simulink model "SA_decouple_angles"  (R2016a)
settings: Solver=ode45  StartTime=0.0  StopTime=tfin  FixedStep=0.001  RelTol=1e-09
values from neighbouring files (symbols this model uses):
  den_av_SA91 = [1 -p_av_SA91]    [SA_9.m]    (also in SA_9cas1.m)
  den_AvPh_SA8 = [1 -p]    [SA_8.m]
  den_PI_SA8 = [1 -p]    [SA_8.m]
  den_re_SA91 = [1 -p_re_SA91]    [SA_9.m]    (also in SA_9cas1.m)
  Ka_av_SA91 = K_des/alf    [SA_9.m]    (also in SA_9cas1.m)
  Ka_SA8 = abs((polyval(den_phi,pdes)*polyval(den_AvPh_SA8,pdes)*polyval(den_PI_SA8,pdes))/(polyval(num_AvPh_SA8,pdes)*polyval(num_phi,pdes)*polyval(num_PI_SA8,pdes)))    [SA_8.m]
  Kp_XX = -z*Kv_XX    [SA_10.m]    (also in SA_10x.m; SA_10y.m)
  Kp_YY = -z*Kv_YY    [SA_10y.m]
  Kr_SA91 = K_des/beta    [SA_9.m]    (also in SA_9cas1.m)
  Kv_XX = 1/abs(polyval(conv(num_a_XX,num_Sx(1,:)),p_des)/polyval(conv(den_a_XX,den_Sx),p_des))    [SA_10.m]    (also in SA_10x.m; SA_10y.m)
  Kv_YY = 1/abs(polyval(conv(num_a_YY,num_Sy(1,:)),p_des)/polyval(conv(den_a_YY,den_Sy),p_des))    [SA_10y.m]
  num_av_SA91 = [1 -z_av_SA91]    [SA_9.m]    (also in SA_9cas1.m)
  num_AvPh_SA8 = [1 -z]    [SA_8.m]
  num_PI_SA8 = [1 -z]    [SA_8.m]
  num_re_SA91 = [1 -z_re_SA91]    [SA_9.m]    (also in SA_9cas1.m)
undefined symbols (not defined in the file or in its folder): A_phi, A_theta, A_z, ae0, ae1, ae2, ae3, as0, as1, as2, as3, AxS, AyS, B_phi, B_theta, B_z, be1, BxS, ByS, C3_3_iden, CxS, CyS, D_phi, D_theta, D_z, DxS, DyS, ia_e, ib_e, ic_e, phi_e, TABC_trans, TDEF_trans, theta_e, U, U_inv, va_e, vb_e, vc_e, vx_s_e, vy_s_e, vz_e, w_phi_e, w_theta_e, x_s_e, y_s_e, z_e
libraries: simulink_extras x3
settings Model: Creator=delafontaine  LastModifiedBy=genp2203
settings SolverCC: AlgebraicLoopSolver=LineSearch
settings DataIOCC: LimitDataPoints=on  SaveFormat=Array  SignalLoggingSaveFormat=ModelDataLogs
settings DebuggingCC: UnderspecifiedInitializationDetection=Classic  MergeDetectMultiDrivingBlocksExec=none  MultiTaskDSMMsg=warning  MultiTaskCondExecSysMsg=none
settings HardwareCC: ProdBitPerPointer=32  ProdLargestAtomicFloat=None  ProdIntDivRoundTo=Undefined  ProdEndianess=Unspecified  ProdWordSize=32  ProdHWDeviceType=32-bit Generic
settings ModelReferenceCC: PropagateSignalLabelsOutOfModel=off
settings ConfigComp: CovModelRefEnable=Off  CovSFcnEnable=off

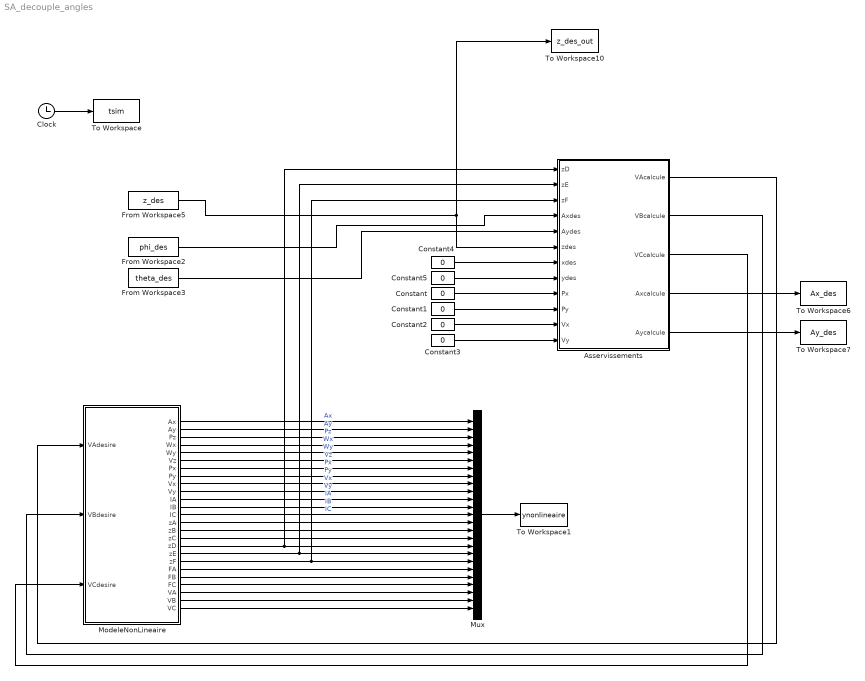
== system SA_decouple_angles ==
  Asservissements : Subsystem
      mask help: Simulink:masks:GenSFuncDesc_MD
      mask Help: eval('feval(''rtwprivate'',''rtwhelpview'',''rtw_sfcn_block'')');
  Clock : Clock
  Constant{,1..5} (6 alike) : Constant  Value=0
  From Workspace2 : FromWorkspace  VariableName=phi_des  SampleTime=0  Interpolate=off  OutputAfterFinalValue=Holding final value
  From Workspace3 : FromWorkspace  VariableName=theta_des  SampleTime=0  Interpolate=off  OutputAfterFinalValue=Holding final value
  From Workspace5 : FromWorkspace  VariableName=z_des  SampleTime=0  Interpolate=off  OutputAfterFinalValue=Holding final value
  ModeleNonLineaire : Subsystem
      mask help: Simulink:masks:GenSFuncDesc_MD
      mask Help: eval('feval(''rtwprivate'',''rtwhelpview'',''rtw_sfcn_block'')');
  Mux : Mux  Inputs=25
  To Workspace : ToWorkspace  VariableName=tsim  SampleTime=-1
  To Workspace1 : ToWorkspace  VariableName=ynonlineaire  SampleTime=-1
  To Workspace10 : ToWorkspace  VariableName=z_des_out  SampleTime=-1
  To Workspace6 : ToWorkspace  VariableName=Ax_des  SampleTime=-1
  To Workspace7 : ToWorkspace  VariableName=Ay_des  SampleTime=-1
  wires:
  Mux/1 -> To Workspace1/1
  Clock/1 -> To Workspace/1
  From Workspace5/1 -> Asservissements/6(zdes), To Workspace10/1
  ModeleNonLineaire/1(Ax) -> Mux/1  "Ax"
  ModeleNonLineaire/2(Ay) -> Mux/2  "Ay"
  ModeleNonLineaire/3(Pz) -> Mux/3  "Pz"
  ModeleNonLineaire/4(Wx) -> Mux/4  "Wx"
  ModeleNonLineaire/5(Wy) -> Mux/5  "Wy"
  ModeleNonLineaire/6(Vz) -> Mux/6  "Vz"
  ModeleNonLineaire/7(Px) -> Mux/7  "Px"
  ModeleNonLineaire/8(Py) -> Mux/8  "Py"
  ModeleNonLineaire/9(Vx) -> Mux/9  "Vx"
  ModeleNonLineaire/10(Vy) -> Mux/10  "Vy"
  ModeleNonLineaire/11(IA) -> Mux/11  "IA"
  ModeleNonLineaire/12(IB) -> Mux/12  "IB"
  ModeleNonLineaire/13(IC) -> Mux/13  "IC"
  ModeleNonLineaire/20(FA) -> Mux/20
  ModeleNonLineaire/21(FB) -> Mux/21
  ModeleNonLineaire/22(FC) -> Mux/22
  ModeleNonLineaire/23(VA) -> Mux/23
  ModeleNonLineaire/24(VB) -> Mux/24
  ModeleNonLineaire/25(VC) -> Mux/25
  ModeleNonLineaire/17(zD) -> Asservissements/1(zD), Mux/17
  ModeleNonLineaire/18(zE) -> Asservissements/2(zE), Mux/18
  ModeleNonLineaire/19(zF) -> Asservissements/3(zF), Mux/19
  ModeleNonLineaire/14(zA) -> Mux/14
  ModeleNonLineaire/15(zB) -> Mux/15
  ModeleNonLineaire/16(zC) -> Mux/16
  Asservissements/4(Axcalcule) -> To Workspace6/1
  Asservissements/5(Aycalcule) -> To Workspace7/1
  Asservissements/1(VAcalcule) -> ModeleNonLineaire/1(VAdesire)
  Asservissements/2(VBcalcule) -> ModeleNonLineaire/2(VBdesire)
  Asservissements/3(VCcalcule) -> ModeleNonLineaire/3(VCdesire)
  Constant/1 -> Asservissements/9(Px)
  Constant1/1 -> Asservissements/10(Py)
  Constant2/1 -> Asservissements/11(Vx)
  Constant3/1 -> Asservissements/12(Vy)
  From Workspace2/1 -> Asservissements/4(Axdes)
  From Workspace3/1 -> Asservissements/5(Aydes)
  Constant4/1 -> Asservissements/7(xdes)
  Constant5/1 -> Asservissements/8(ydes)

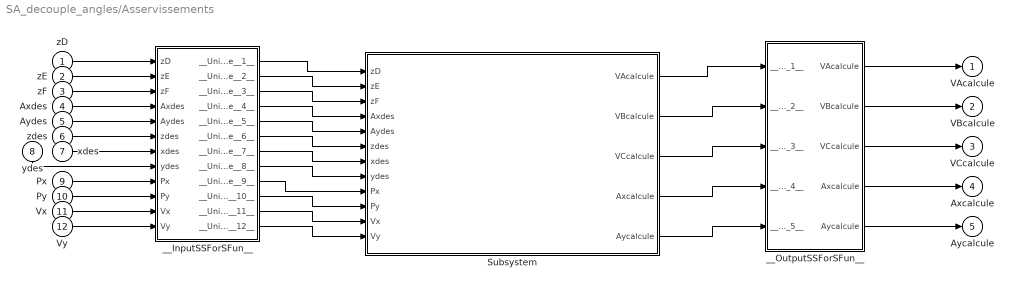
== system SA_decouple_angles/Asservissements ==
  zD : Inport
  zE : Inport  Port=2
  zF : Inport  Port=3
  Axdes : Inport  Port=4
  Aydes : Inport  Port=5
  zdes : Inport  Port=6
  xdes : Inport  Port=7
  ydes : Inport  Port=8
  Px : Inport  Port=9
  Py : Inport  Port=10
  Vx : Inport  Port=11
  Vy : Inport  Port=12
  Subsystem : Subsystem
  __InputSSForSFun__ : Subsystem
  __OutputSSForSFun__ : Subsystem
  VAcalcule : Outport
  VBcalcule : Outport  Port=2
  VCcalcule : Outport  Port=3
  Axcalcule : Outport  Port=4
  Aycalcule : Outport  Port=5
  wires:
  zD/1 -> __InputSSForSFun__/1(zD)
  zE/1 -> __InputSSForSFun__/2(zE)
  zF/1 -> __InputSSForSFun__/3(zF)
  Axdes/1 -> __InputSSForSFun__/4(Axdes)
  Aydes/1 -> __InputSSForSFun__/5(Aydes)
  zdes/1 -> __InputSSForSFun__/6(zdes)
  xdes/1 -> __InputSSForSFun__/7(xdes)
  ydes/1 -> __InputSSForSFun__/8(ydes)
  Px/1 -> __InputSSForSFun__/9(Px)
  Py/1 -> __InputSSForSFun__/10(Py)
  Vx/1 -> __InputSSForSFun__/11(Vx)
  Vy/1 -> __InputSSForSFun__/12(Vy)
  __InputSSForSFun__/1(__UniqueOutportName__1__) -> Subsystem/1(zD)
  __InputSSForSFun__/2(__UniqueOutportName__2__) -> Subsystem/2(zE)
  __InputSSForSFun__/3(__UniqueOutportName__3__) -> Subsystem/3(zF)
  __InputSSForSFun__/4(__UniqueOutportName__4__) -> Subsystem/4(Axdes)
  __InputSSForSFun__/5(__UniqueOutportName__5__) -> Subsystem/5(Aydes)
  __InputSSForSFun__/6(__UniqueOutportName__6__) -> Subsystem/6(zdes)
  __InputSSForSFun__/7(__UniqueOutportName__7__) -> Subsystem/7(xdes)
  __InputSSForSFun__/8(__UniqueOutportName__8__) -> Subsystem/8(ydes)
  __InputSSForSFun__/9(__UniqueOutportName__9__) -> Subsystem/9(Px)
  __InputSSForSFun__/10(__UniqueOutportName__10__) -> Subsystem/10(Py)
  __InputSSForSFun__/11(__UniqueOutportName__11__) -> Subsystem/11(Vx)
  __InputSSForSFun__/12(__UniqueOutportName__12__) -> Subsystem/12(Vy)
  Subsystem/1(VAcalcule) -> __OutputSSForSFun__/1(__UniqueInportName__1__)
  Subsystem/2(VBcalcule) -> __OutputSSForSFun__/2(__UniqueInportName__2__)
  Subsystem/3(VCcalcule) -> __OutputSSForSFun__/3(__UniqueInportName__3__)
  Subsystem/4(Axcalcule) -> __OutputSSForSFun__/4(__UniqueInportName__4__)
  Subsystem/5(Aycalcule) -> __OutputSSForSFun__/5(__UniqueInportName__5__)
  __OutputSSForSFun__/1(VAcalcule) -> VAcalcule/1
  __OutputSSForSFun__/2(VBcalcule) -> VBcalcule/1
  __OutputSSForSFun__/3(VCcalcule) -> VCcalcule/1
  __OutputSSForSFun__/4(Axcalcule) -> Axcalcule/1
  __OutputSSForSFun__/5(Aycalcule) -> Aycalcule/1

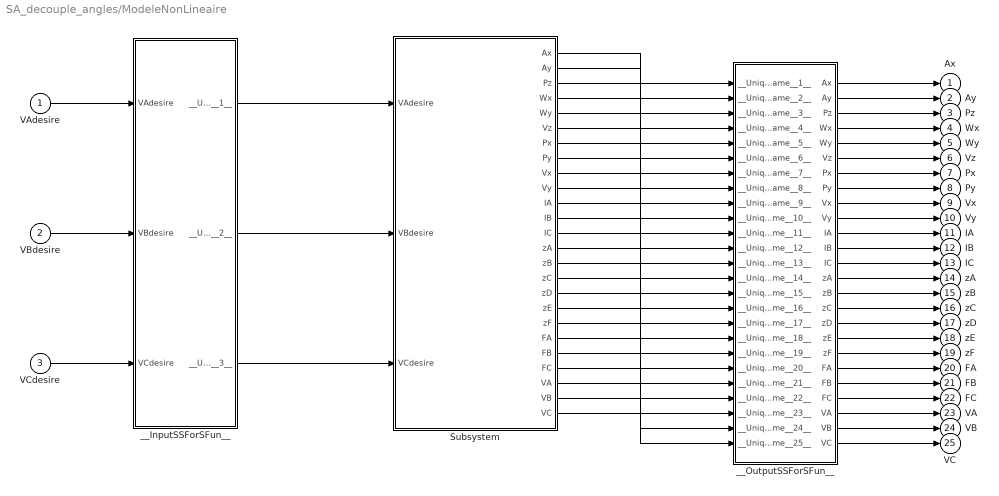
== system SA_decouple_angles/ModeleNonLineaire ==
  VAdesire : Inport
  VBdesire : Inport  Port=2
  VCdesire : Inport  Port=3
  Subsystem : Subsystem
  __InputSSForSFun__ : Subsystem
  __OutputSSForSFun__ : Subsystem
  Ax : Outport
  Ay : Outport  Port=2
  Pz : Outport  Port=3
  Wx : Outport  Port=4
  Wy : Outport  Port=5
  Vz : Outport  Port=6
  Px : Outport  Port=7
  Py : Outport  Port=8
  Vx : Outport  Port=9
  Vy : Outport  Port=10
  IA : Outport  Port=11
  IB : Outport  Port=12
  IC : Outport  Port=13
  zA : Outport  Port=14
  zB : Outport  Port=15
  zC : Outport  Port=16
  zD : Outport  Port=17
  zE : Outport  Port=18
  zF : Outport  Port=19
  FA : Outport  Port=20
  FB : Outport  Port=21
  FC : Outport  Port=22
  VA : Outport  Port=23
  VB : Outport  Port=24
  VC : Outport  Port=25
  wires:
  VAdesire/1 -> __InputSSForSFun__/1(VAdesire)
  VBdesire/1 -> __InputSSForSFun__/2(VBdesire)
  VCdesire/1 -> __InputSSForSFun__/3(VCdesire)
  __InputSSForSFun__/1(__UniqueOutportName__1__) -> Subsystem/1(VAdesire)
  __InputSSForSFun__/2(__UniqueOutportName__2__) -> Subsystem/2(VBdesire)
  __InputSSForSFun__/3(__UniqueOutportName__3__) -> Subsystem/3(VCdesire)
  Subsystem/1(Ax) -> __OutputSSForSFun__/1(__UniqueInportName__1__)
  Subsystem/2(Ay) -> __OutputSSForSFun__/2(__UniqueInportName__2__)
  Subsystem/3(Pz) -> __OutputSSForSFun__/3(__UniqueInportName__3__)
  Subsystem/4(Wx) -> __OutputSSForSFun__/4(__UniqueInportName__4__)
  Subsystem/5(Wy) -> __OutputSSForSFun__/5(__UniqueInportName__5__)
  Subsystem/6(Vz) -> __OutputSSForSFun__/6(__UniqueInportName__6__)
  Subsystem/7(Px) -> __OutputSSForSFun__/7(__UniqueInportName__7__)
  Subsystem/8(Py) -> __OutputSSForSFun__/8(__UniqueInportName__8__)
  Subsystem/9(Vx) -> __OutputSSForSFun__/9(__UniqueInportName__9__)
  Subsystem/10(Vy) -> __OutputSSForSFun__/10(__UniqueInportName__10__)
  Subsystem/11(IA) -> __OutputSSForSFun__/11(__UniqueInportName__11__)
  Subsystem/12(IB) -> __OutputSSForSFun__/12(__UniqueInportName__12__)
  Subsystem/13(IC) -> __OutputSSForSFun__/13(__UniqueInportName__13__)
  Subsystem/14(zA) -> __OutputSSForSFun__/14(__UniqueInportName__14__)
  Subsystem/15(zB) -> __OutputSSForSFun__/15(__UniqueInportName__15__)
  Subsystem/16(zC) -> __OutputSSForSFun__/16(__UniqueInportName__16__)
  Subsystem/17(zD) -> __OutputSSForSFun__/17(__UniqueInportName__17__)
  Subsystem/18(zE) -> __OutputSSForSFun__/18(__UniqueInportName__18__)
  Subsystem/19(zF) -> __OutputSSForSFun__/19(__UniqueInportName__19__)
  Subsystem/20(FA) -> __OutputSSForSFun__/20(__UniqueInportName__20__)
  Subsystem/21(FB) -> __OutputSSForSFun__/21(__UniqueInportName__21__)
  Subsystem/22(FC) -> __OutputSSForSFun__/22(__UniqueInportName__22__)
  Subsystem/23(VA) -> __OutputSSForSFun__/23(__UniqueInportName__23__)
  Subsystem/24(VB) -> __OutputSSForSFun__/24(__UniqueInportName__24__)
  Subsystem/25(VC) -> __OutputSSForSFun__/25(__UniqueInportName__25__)
  __OutputSSForSFun__/1(Ax) -> Ax/1
  __OutputSSForSFun__/2(Ay) -> Ay/1
  __OutputSSForSFun__/3(Pz) -> Pz/1
  __OutputSSForSFun__/4(Wx) -> Wx/1
  __OutputSSForSFun__/5(Wy) -> Wy/1
  __OutputSSForSFun__/6(Vz) -> Vz/1
  __OutputSSForSFun__/7(Px) -> Px/1
  __OutputSSForSFun__/8(Py) -> Py/1
  __OutputSSForSFun__/9(Vx) -> Vx/1
  __OutputSSForSFun__/10(Vy) -> Vy/1
  __OutputSSForSFun__/11(IA) -> IA/1
  __OutputSSForSFun__/12(IB) -> IB/1
  __OutputSSForSFun__/13(IC) -> IC/1
  __OutputSSForSFun__/14(zA) -> zA/1
  __OutputSSForSFun__/15(zB) -> zB/1
  __OutputSSForSFun__/16(zC) -> zC/1
  __OutputSSForSFun__/17(zD) -> zD/1
  __OutputSSForSFun__/18(zE) -> zE/1
  __OutputSSForSFun__/19(zF) -> zF/1
  __OutputSSForSFun__/20(FA) -> FA/1
  __OutputSSForSFun__/21(FB) -> FB/1
  __OutputSSForSFun__/22(FC) -> FC/1
  __OutputSSForSFun__/23(VA) -> VA/1
  __OutputSSForSFun__/24(VB) -> VB/1
  __OutputSSForSFun__/25(VC) -> VC/1

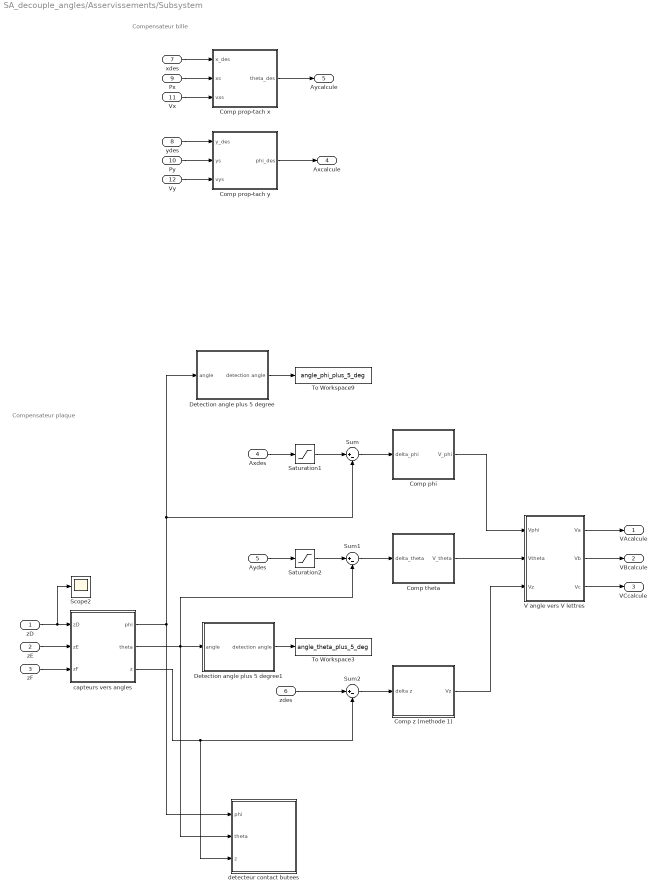
== system SA_decouple_angles/Asservissements/Subsystem ==
  note: Compensateur plaque
  note: Compensateur bille
  zD : Inport
  zE : Inport  Port=2
  zF : Inport  Port=3
  Axdes : Inport  Port=4
  Aydes : Inport  Port=5
  zdes : Inport  Port=6
  xdes : Inport  Port=7
  ydes : Inport  Port=8
  Px : Inport  Port=9
  Py : Inport  Port=10
  Vx : Inport  Port=11
  Vy : Inport  Port=12
  Comp phi : Subsystem
  Comp prop-tach x : Subsystem
  Comp prop-tach y : Subsystem
  Comp theta : Subsystem
  Comp z (methode 1) : Subsystem
  Detection angle plus 5 degree : Subsystem
  Detection angle plus 5 degree1 : Subsystem
  Saturation1 : Saturate  UpperLimit=deg2rad(5)  LowerLimit=deg2rad(-5)
  Saturation2 : Saturate  UpperLimit=deg2rad(5)  LowerLimit=deg2rad(-5)
  Scope2 : Scope
  Sum : Sum  Inputs=|+-
  Sum1 : Sum  Inputs=|+-
  Sum2 : Sum  Inputs=|+-
  To Workspace3 : ToWorkspace  VariableName=angle_theta_plus_5_deg  SampleTime=-1
      settings: MaxDataPoints=1
  To Workspace9 : ToWorkspace  VariableName=angle_phi_plus_5_deg  SampleTime=-1
      settings: MaxDataPoints=1
  V angle vers V lettres : Subsystem
  capteurs vers angles : Subsystem
  detecteur contact butees : Subsystem
  VAcalcule : Outport
  VBcalcule : Outport  Port=2
  VCcalcule : Outport  Port=3
  Axcalcule : Outport  Port=4
  Aycalcule : Outport  Port=5
  wires:
  Sum/1 -> Comp phi/1(delta_phi)
  ydes/1 -> Comp prop-tach y/1(y_des)
  xdes/1 -> Comp prop-tach x/1(x_des)
  Vx/1 -> Comp prop-tach x/3(vxs)
  Px/1 -> Comp prop-tach x/2(xs)
  Py/1 -> Comp prop-tach y/2(ys)
  Vy/1 -> Comp prop-tach y/3(vys)
  zD/1 -> Scope2/1, capteurs vers angles/1(zD)
  zE/1 -> capteurs vers angles/2(zE)
  zF/1 -> capteurs vers angles/3(zF)
  capteurs vers angles/1(phi) -> Sum/2, Detection angle plus 5 degree/1(angle), detecteur contact butees/1(phi)
  V angle vers V lettres/3(Vc) -> VCcalcule/1
  V angle vers V lettres/2(Vb) -> VBcalcule/1
  V angle vers V lettres/1(Va) -> VAcalcule/1
  Comp phi/1(V_phi) -> V angle vers V lettres/1(Vphi)
  Comp theta/1(V_theta) -> V angle vers V lettres/2(Vtheta)
  Sum1/1 -> Comp theta/1(delta_theta)
  capteurs vers angles/3(z) -> detecteur contact butees/3(z), Sum2/2
  zdes/1 -> Sum2/1
  Sum2/1 -> Comp z (methode 1)/1(delta z)
  Comp prop-tach y/1(phi_des) -> Axcalcule/1
  Comp prop-tach x/1(theta_des) -> Aycalcule/1
  Comp z (methode 1)/1(Vz) -> V angle vers V lettres/3(Vz)
  Detection angle plus 5 degree/1(detection angle) -> To Workspace9/1
  Detection angle plus 5 degree1/1(detection angle) -> To Workspace3/1
  capteurs vers angles/2(theta) -> Detection angle plus 5 degree1/1(angle), Sum1/2, detecteur contact butees/2(theta)
  Axdes/1 -> Saturation1/1
  Saturation1/1 -> Sum/1
  Saturation2/1 -> Sum1/1
  Aydes/1 -> Saturation2/1

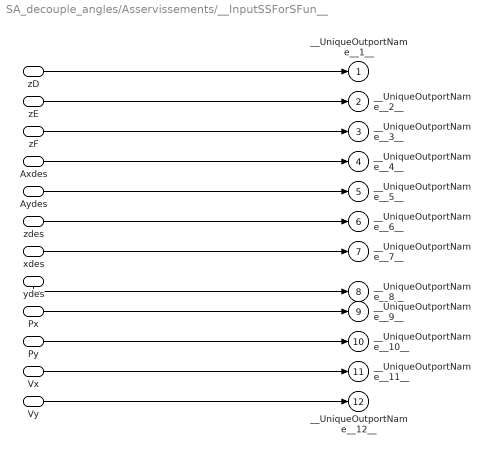
== system SA_decouple_angles/Asservissements/__InputSSForSFun__ ==
  zD : Inport
  zE : Inport  Port=2
  zF : Inport  Port=3
  Axdes : Inport  Port=4
  Aydes : Inport  Port=5
  zdes : Inport  Port=6
  xdes : Inport  Port=7
  ydes : Inport  Port=8
  Px : Inport  Port=9
  Py : Inport  Port=10
  Vx : Inport  Port=11
  Vy : Inport  Port=12
  __UniqueOutportName__1__ : Outport
  __UniqueOutportName__2__ : Outport  Port=2
  __UniqueOutportName__3__ : Outport  Port=3
  __UniqueOutportName__4__ : Outport  Port=4
  __UniqueOutportName__5__ : Outport  Port=5
  __UniqueOutportName__6__ : Outport  Port=6
  __UniqueOutportName__7__ : Outport  Port=7
  __UniqueOutportName__8__ : Outport  Port=8
  __UniqueOutportName__9__ : Outport  Port=9
  __UniqueOutportName__10__ : Outport  Port=10
  __UniqueOutportName__11__ : Outport  Port=11
  __UniqueOutportName__12__ : Outport  Port=12
  wires:
  zD/1 -> __UniqueOutportName__1__/1
  zE/1 -> __UniqueOutportName__2__/1
  zF/1 -> __UniqueOutportName__3__/1
  Axdes/1 -> __UniqueOutportName__4__/1
  Aydes/1 -> __UniqueOutportName__5__/1
  zdes/1 -> __UniqueOutportName__6__/1
  xdes/1 -> __UniqueOutportName__7__/1
  ydes/1 -> __UniqueOutportName__8__/1
  Px/1 -> __UniqueOutportName__9__/1
  Py/1 -> __UniqueOutportName__10__/1
  Vx/1 -> __UniqueOutportName__11__/1
  Vy/1 -> __UniqueOutportName__12__/1

== system SA_decouple_angles/Asservissements/__OutputSSForSFun__ ==
  __UniqueInportName__1__ : Inport
  __UniqueInportName__2__ : Inport  Port=2
  __UniqueInportName__3__ : Inport  Port=3
  __UniqueInportName__4__ : Inport  Port=4
  __UniqueInportName__5__ : Inport  Port=5
  VAcalcule : Outport
  VBcalcule : Outport  Port=2
  VCcalcule : Outport  Port=3
  Axcalcule : Outport  Port=4
  Aycalcule : Outport  Port=5
  wires:
  __UniqueInportName__1__/1 -> VAcalcule/1
  __UniqueInportName__2__/1 -> VBcalcule/1
  __UniqueInportName__3__/1 -> VCcalcule/1
  __UniqueInportName__4__/1 -> Axcalcule/1  "Ax_des"
  __UniqueInportName__5__/1 -> Aycalcule/1  "Ay_des"

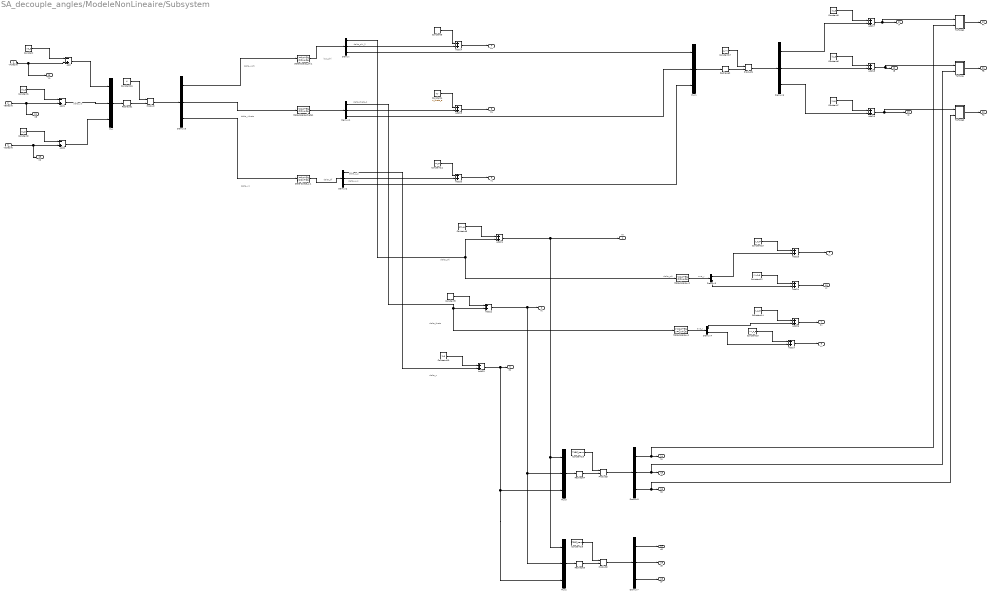
== system SA_decouple_angles/ModeleNonLineaire/Subsystem ==
  note: axe_x
  note: axe_y
  note: delta_phi
  note: delta_w_z
  note: delta_z_2
  note: delta_theta_2
  note: delta_phi_2
  note: delta_phi
  note: delta_vb
  note: delta_z
  note: delta_theta
  note: bus_phi
  note: delat_df
  note: delta_vphi
  note: delta_vtheta
  note: delta_vz
  VAdesire : Inport
  VBdesire : Inport  Port=2
  VCdesire : Inport  Port=3
  Add : Sum  Inputs=-+
  Add1 : Sum  Inputs=-+
  Add{13..14,17..27} (13 alike) : Sum
  Add2 : Sum  Inputs=-+
  Constant : Constant  Value=va_e
  Constant1 : Constant  Value=vb_e
  Constant10 : Constant  Value=z_e
  Constant11 : Constant  Value=vz_e
  Constant12 : Constant  Value=vy_s_e
  Constant13 : Constant  Value=y_s_e
  Constant14 : Constant  Value=x_s_e
  Constant15 : Constant  Value=vx_s_e
  Constant16 : Constant  Value=U  VectorParams1D=off
  Constant17 : Constant  Value=U_inv  VectorParams1D=off
  Constant18 : Constant  Value=TDEF_trans  VectorParams1D=off
  Constant19 : Constant  Value=TABC_trans  VectorParams1D=off
  Constant2 : Constant  Value=vc_e
  Constant3 : Constant  Value=ia_e
  Constant4 : Constant  Value=w_theta_e
  Constant5 : Constant  Value=w_phi_e
  Constant6 : Constant  Value=ib_e
  Constant7 : Constant  Value=ic_e
  Constant8 : Constant  Value=phi_e
  Constant9 : Constant  Value=theta_e
  Demux{,1..2,5..8} (7 alike) : Demux  Outputs=3
  Demux3 : Demux  Outputs=2
  Demux4 : Demux  Outputs=2
  Mux{,1..3} (4 alike) : Mux  Inputs=3
  Product{,1..3} (4 alike) : Product  Multiplication=Matrix(*)
  Reshape{1..4} (4 alike) : Reshape  OutputDimensionality=Column vector (2-D)  OutputDimensions=[3:1]
  State-Space_phi1 : StateSpace  A=A_phi  B=B_phi  C=C3_3_iden  D=D_phi  X0=0
  State-Space_theta1 : StateSpace  A=A_theta  B=B_theta  C=C3_3_iden  D=D_theta  X0=0
  State-Space_xs : StateSpace  A=AyS  B=ByS  C=CyS  D=DyS  X0=0
  State-Space_ys : StateSpace  A=AxS  B=BxS  C=CxS  D=DxS  X0=0
  State-Space_z 1 : StateSpace  A=A_z  B=B_z  C=C3_3_iden  D=D_z  X0=0
  ToForce : Subsystem
  ToForce1 : Subsystem
  ToForce2 : Subsystem
  Ax : Outport
  Ay : Outport  Port=2
  Pz : Outport  Port=3
  Wx : Outport  Port=4
  Wy : Outport  Port=5
  Vz : Outport  Port=6
  Px : Outport  Port=7
  Py : Outport  Port=8
  Vx : Outport  Port=9
  Vy : Outport  Port=10
  IA : Outport  Port=11
  IB : Outport  Port=12
  IC : Outport  Port=13
  zA : Outport  Port=14
  zB : Outport  Port=15
  zC : Outport  Port=16
  zD : Outport  Port=17
  zE : Outport  Port=18
  zF : Outport  Port=19
  FA : Outport  Port=20
  FB : Outport  Port=21
  FC : Outport  Port=22
  VA : Outport  Port=23
  VB : Outport  Port=24
  VC : Outport  Port=25
  wires:
  Constant/1 -> Add/1
  VAdesire/1 -> VA/1, Add/2
  Constant2/1 -> Add2/1
  VCdesire/1 -> VC/1, Add2/2
  Constant1/1 -> Add1/1
  VBdesire/1 -> VB/1, Add1/2
  Demux2/1 -> Add23/2
  Demux5/1 -> State-Space_phi1/1
  Demux5/2 -> State-Space_theta1/1
  Demux5/3 -> State-Space_z 1/1
  State-Space_phi1/1 -> Demux/1
  State-Space_theta1/1 -> Demux1/1  "delta_de"
  State-Space_z 1/1 -> Demux2/1
  Demux1/2 -> Add13/2  "delta_w_theta"
  Demux2/2 -> Add20/2
  Constant4/1 -> Add13/1
  Constant5/1 -> Add14/1
  Constant11/1 -> Add20/1
  Add14/1 -> Wx/1
  Add13/1 -> Wy/1
  Add20/1 -> Vz/1
  Demux/3 -> Mux1/1  "delta_i_phi"
  Demux1/3 -> Mux1/2  "delta_i_theta"
  Demux2/3 -> Mux1/3  "delta_i_z"
  Constant3/1 -> Add17/1
  Constant6/1 -> Add18/1
  Constant7/1 -> Add19/1
  Constant8/1 -> Add21/1
  Constant9/1 -> Add22/1
  Constant10/1 -> Add23/1
  Demux/1 -> Add21/2, State-Space_xs/1
  State-Space_xs/1 -> Demux3/1
  Demux1/1 -> State-Space_ys/1, Add22/2  "delta_theta"
  State-Space_ys/1 -> Demux4/1
  Demux3/1 -> Add25/2  "delta_ys"
  Demux3/2 -> Add24/2  "dela_vys"
  Demux4/1 -> Add26/2  "delta_xs"
  Demux4/2 -> Add27/2  "delta_vxs"
  Constant12/1 -> Add24/1
  Constant13/1 -> Add25/1
  Constant14/1 -> Add26/1
  Constant15/1 -> Add27/1
  Add25/1 -> Py/1
  Add24/1 -> Vy/1
  Add26/1 -> Px/1
  Add27/1 -> Vx/1
  Demux7/1 -> zD/1
  Add21/1 -> Mux3/1, Mux2/1, Ax/1  "phi"
  Demux7/2 -> zE/1
  Add22/1 -> Mux3/2, Mux2/2, Ay/1  "theta"
  Add23/1 -> Mux3/3, Mux2/3, Pz/1  "z"
  Demux7/3 -> zF/1
  Add17/1 -> ToForce1/1(I), IA/1
  Add18/1 -> IB/1, ToForce/1(I)
  Add19/1 -> ToForce2/1(I), IC/1
  ToForce/1(Force) -> FB/1
  ToForce1/1(Force) -> FA/1
  ToForce2/1(Force) -> FC/1
  Add/1 -> Mux/1  "delta_va"
  Add1/1 -> Mux/2  "delta_vb"
  Add2/1 -> Mux/3  "delta_vc"
  Constant16/1 -> Product/1
  Product/1 -> Demux5/1
  Mux/1 -> Reshape1/1
  Reshape1/1 -> Product/2
  Constant17/1 -> Product1/1
  Product1/1 -> Demux6/1
  Mux1/1 -> Reshape2/1
  Reshape2/1 -> Product1/2
  Demux6/1 -> Add17/2
  Demux6/2 -> Add18/2
  Demux6/3 -> Add19/2
  Demux/2 -> Add14/2  "delta_w_phi"
  Constant18/1 -> Product2/1
  Product2/1 -> Demux7/1
  Mux2/1 -> Reshape3/1
  Reshape3/1 -> Product2/2
  Constant19/1 -> Product3/1
  Product3/1 -> Demux8/1
  Mux3/1 -> Reshape4/1
  Reshape4/1 -> Product3/2
  Demux8/3 -> ToForce2/2(Z), zC/1
  Demux8/2 -> zB/1, ToForce/2(Z)
  Demux8/1 -> ToForce1/2(Z), zA/1

== system SA_decouple_angles/ModeleNonLineaire/__InputSSForSFun__ ==
  VAdesire : Inport
  VBdesire : Inport  Port=2
  VCdesire : Inport  Port=3
  __UniqueOutportName__1__ : Outport
  __UniqueOutportName__2__ : Outport  Port=2
  __UniqueOutportName__3__ : Outport  Port=3
  wires:
  VAdesire/1 -> __UniqueOutportName__1__/1
  VBdesire/1 -> __UniqueOutportName__2__/1
  VCdesire/1 -> __UniqueOutportName__3__/1

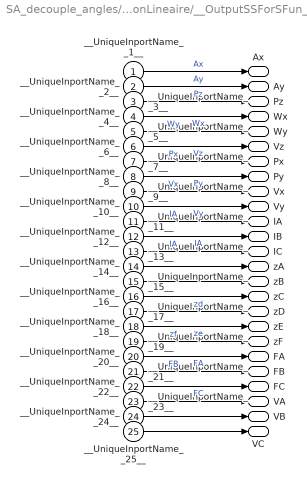
== system SA_decouple_angles/ModeleNonLineaire/__OutputSSForSFun__ ==
  __UniqueInportName__1__ : Inport
  __UniqueInportName__2__ : Inport  Port=2
  __UniqueInportName__3__ : Inport  Port=3
  __UniqueInportName__4__ : Inport  Port=4
  __UniqueInportName__5__ : Inport  Port=5
  __UniqueInportName__6__ : Inport  Port=6
  __UniqueInportName__7__ : Inport  Port=7
  __UniqueInportName__8__ : Inport  Port=8
  __UniqueInportName__9__ : Inport  Port=9
  __UniqueInportName__10__ : Inport  Port=10
  __UniqueInportName__11__ : Inport  Port=11
  __UniqueInportName__12__ : Inport  Port=12
  __UniqueInportName__13__ : Inport  Port=13
  __UniqueInportName__14__ : Inport  Port=14
  __UniqueInportName__15__ : Inport  Port=15
  __UniqueInportName__16__ : Inport  Port=16
  __UniqueInportName__17__ : Inport  Port=17
  __UniqueInportName__18__ : Inport  Port=18
  __UniqueInportName__19__ : Inport  Port=19
  __UniqueInportName__20__ : Inport  Port=20
  __UniqueInportName__21__ : Inport  Port=21
  __UniqueInportName__22__ : Inport  Port=22
  __UniqueInportName__23__ : Inport  Port=23
  __UniqueInportName__24__ : Inport  Port=24
  __UniqueInportName__25__ : Inport  Port=25
  Ax : Outport
  Ay : Outport  Port=2
  Pz : Outport  Port=3
  Wx : Outport  Port=4
  Wy : Outport  Port=5
  Vz : Outport  Port=6
  Px : Outport  Port=7
  Py : Outport  Port=8
  Vx : Outport  Port=9
  Vy : Outport  Port=10
  IA : Outport  Port=11
  IB : Outport  Port=12
  IC : Outport  Port=13
  zA : Outport  Port=14
  zB : Outport  Port=15
  zC : Outport  Port=16
  zD : Outport  Port=17
  zE : Outport  Port=18
  zF : Outport  Port=19
  FA : Outport  Port=20
  FB : Outport  Port=21
  FC : Outport  Port=22
  VA : Outport  Port=23
  VB : Outport  Port=24
  VC : Outport  Port=25
  wires:
  __UniqueInportName__1__/1 -> Ax/1  "Ax"
  __UniqueInportName__2__/1 -> Ay/1  "Ay"
  __UniqueInportName__3__/1 -> Pz/1  "Pz"
  __UniqueInportName__4__/1 -> Wx/1  "Wx"
  __UniqueInportName__5__/1 -> Wy/1  "Wy"
  __UniqueInportName__6__/1 -> Vz/1  "Vz"
  __UniqueInportName__7__/1 -> Px/1  "Px"
  __UniqueInportName__8__/1 -> Py/1  "Py"
  __UniqueInportName__9__/1 -> Vx/1  "Vx"
  __UniqueInportName__10__/1 -> Vy/1  "Vy"
  __UniqueInportName__11__/1 -> IA/1  "IA"
  __UniqueInportName__12__/1 -> IB/1  "IA"
  __UniqueInportName__13__/1 -> IC/1  "IA"
  __UniqueInportName__14__/1 -> zA/1
  __UniqueInportName__15__/1 -> zB/1
  __UniqueInportName__16__/1 -> zC/1
  __UniqueInportName__17__/1 -> zD/1  "zd"
  __UniqueInportName__18__/1 -> zE/1  "ze"
  __UniqueInportName__19__/1 -> zF/1  "zf"
  __UniqueInportName__20__/1 -> FA/1  "FA"
  __UniqueInportName__21__/1 -> FB/1  "FB"
  __UniqueInportName__22__/1 -> FC/1  "FC"
  __UniqueInportName__23__/1 -> VA/1
  __UniqueInportName__24__/1 -> VB/1
  __UniqueInportName__25__/1 -> VC/1

== system SA_decouple_angles/Asservissements/Subsystem/Comp phi ==
  delta_phi : Inport
  Double_AvPh : Subsystem
  PI : TransferFcn  Numerator=num_PI_SA8  Denominator=den_PI_SA8
  V_phi : Outport
  wires:
  PI/1 -> Double_AvPh/1(signal_in)
  delta_phi/1 -> PI/1
  Double_AvPh/1(signal_out) -> V_phi/1

== system SA_decouple_angles/Asservissements/Subsystem/Comp prop-tach x ==
  x_des : Inport
  xs : Inport  Port=2
  vxs : Inport  Port=3
  Gain : Gain  Gain=Kv_XX
  Gain1 : Gain  Gain=Kp_XX
  Sum : Sum  Inputs=|-+
  Sum1 : Sum  Inputs=|++
  theta_des : Outport
  wires:
  Sum/1 -> Gain1/1
  Gain1/1 -> Sum1/1
  Gain/1 -> Sum1/2
  xs/1 -> Sum/2
  vxs/1 -> Gain/1
  Sum1/1 -> theta_des/1
  x_des/1 -> Sum/1

== system SA_decouple_angles/Asservissements/Subsystem/Comp prop-tach y ==
  y_des : Inport
  ys : Inport  Port=2
  vys : Inport  Port=3
  Gain : Gain  Gain=Kv_YY
  Gain1 : Gain  Gain=Kp_YY
  Sum : Sum  Inputs=|+-
  Sum1 : Sum  Inputs=|+-
  phi_des : Outport
  wires:
  Sum/1 -> Gain1/1
  y_des/1 -> Sum/1
  Gain1/1 -> Sum1/1
  Gain/1 -> Sum1/2
  ys/1 -> Sum/2
  vys/1 -> Gain/1
  Sum1/1 -> phi_des/1

== system SA_decouple_angles/Asservissements/Subsystem/Comp theta ==
  delta_theta : Inport
  Double_AvPh : Subsystem
  PI : TransferFcn  Numerator=num_PI_SA8  Denominator=den_PI_SA8
  V_theta : Outport
  wires:
  PI/1 -> Double_AvPh/1(signal_in)
  delta_theta/1 -> PI/1
  Double_AvPh/1(signal_out) -> V_theta/1

== system SA_decouple_angles/Asservissements/Subsystem/Comp z (methode 1) ==
  delta z : Inport
  Double AvPh : Subsystem
  Simple AvPh : Subsystem
  Vz : Outport
  wires:
  delta z/1 -> Double AvPh/1(in)
  Double AvPh/1(out) -> Simple AvPh/1(In1)
  Simple AvPh/1(Out1) -> Vz/1

== system SA_decouple_angles/Asservissements/Subsystem/Detection angle plus 5 degree ==
  angle : Inport
  Constant : Constant  Value=0  OutDataTypeStr=boolean
  Constant1 : Constant  Value=deg2rad(5)  OutDataTypeStr=double
  Constant2 : Constant  Value=deg2rad(-5)  OutDataTypeStr=double
  Logical Operator : Logic  Operator=OR  AllPortsSameDT=off  OutDataTypeStr=boolean
  Relational Operator : RelationalOperator  Operator=>  OutDataTypeStr=boolean
  Relational Operator1 : RelationalOperator  Operator=<  OutDataTypeStr=boolean
  S-R Flip-Flop : simulink_extras/Flip Flops/S-R Flip-Flop  initial_condition=0
  detection angle : Outport
  wires:
  S-R Flip-Flop/1 -> detection angle/1
  angle/1 -> Relational Operator1/1, Relational Operator/1
  Constant1/1 -> Relational Operator/2
  Constant/1 -> S-R Flip-Flop/2
  Constant2/1 -> Relational Operator1/2
  Relational Operator/1 -> Logical Operator/1
  Logical Operator/1 -> S-R Flip-Flop/1
  Relational Operator1/1 -> Logical Operator/2

== system SA_decouple_angles/Asservissements/Subsystem/Detection angle plus 5 degree1 ==
  angle : Inport
  Constant : Constant  Value=0  OutDataTypeStr=boolean
  Constant1 : Constant  Value=deg2rad(5)  OutDataTypeStr=double
  Constant2 : Constant  Value=deg2rad(-5)  OutDataTypeStr=double
  Logical Operator : Logic  Operator=OR  AllPortsSameDT=off  OutDataTypeStr=boolean
  Relational Operator : RelationalOperator  Operator=>  OutDataTypeStr=boolean
  Relational Operator1 : RelationalOperator  Operator=<  OutDataTypeStr=boolean
  S-R Flip-Flop : simulink_extras/Flip Flops/S-R Flip-Flop  initial_condition=0
  detection angle : Outport
  wires:
  S-R Flip-Flop/1 -> detection angle/1
  angle/1 -> Relational Operator1/1, Relational Operator/1
  Constant1/1 -> Relational Operator/2
  Constant/1 -> S-R Flip-Flop/2
  Constant2/1 -> Relational Operator1/2
  Relational Operator/1 -> Logical Operator/1
  Logical Operator/1 -> S-R Flip-Flop/1
  Relational Operator1/1 -> Logical Operator/2

== system SA_decouple_angles/Asservissements/Subsystem/V angle vers V lettres ==
  Vphi : Inport
  Vtheta : Inport  Port=2
  Vz : Inport  Port=3
  Constant : Constant  Value=inv(U)
  Demux : Demux  Outputs=3
  Product : Product  Multiplication=Matrix(*)
  Vector Concatenate : Concatenate  NumInputs=3  Mode=Multidimensional array
  Va : Outport
  Vb : Outport  Port=2
  Vc : Outport  Port=3
  wires:
  Vz/1 -> Vector Concatenate/3
  Vtheta/1 -> Vector Concatenate/2
  Vphi/1 -> Vector Concatenate/1
  Product/1 -> Demux/1
  Constant/1 -> Product/1
  Vector Concatenate/1 -> Product/2
  Demux/3 -> Vc/1
  Demux/2 -> Vb/1
  Demux/1 -> Va/1

== system SA_decouple_angles/Asservissements/Subsystem/capteurs vers angles ==
  zD : Inport
  zE : Inport  Port=2
  zF : Inport  Port=3
  Constant : Constant  Value=inv(TDEF_trans)
  Demux : Demux  Outputs=3
  Product : Product  Multiplication=Matrix(*)
  Vector Concatenate : Concatenate  NumInputs=3  Mode=Multidimensional array
  phi : Outport
  theta : Outport  Port=2
  z : Outport  Port=3
  wires:
  zF/1 -> Vector Concatenate/3
  zE/1 -> Vector Concatenate/2
  zD/1 -> Vector Concatenate/1
  Product/1 -> Demux/1
  Constant/1 -> Product/1
  Vector Concatenate/1 -> Product/2
  Demux/3 -> z/1
  Demux/2 -> theta/1
  Demux/1 -> phi/1

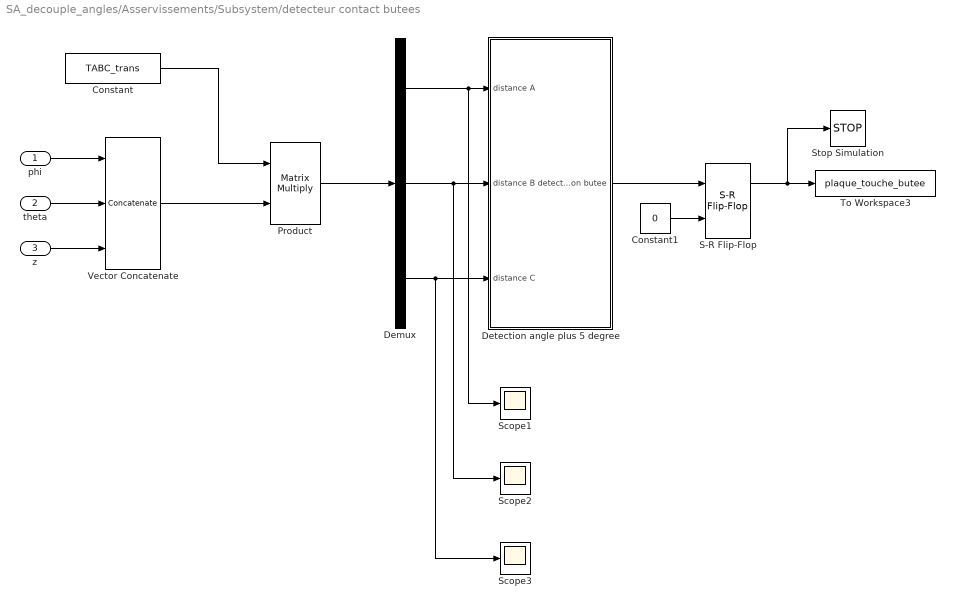
== system SA_decouple_angles/Asservissements/Subsystem/detecteur contact butees ==
  phi : Inport
  theta : Inport  Port=2
  z : Inport  Port=3
  Constant : Constant  Value=TABC_trans
  Constant1 : Constant  Value=0  OutDataTypeStr=boolean
  Demux : Demux  Outputs=3
  Detection angle plus 5 degree : Subsystem
  Product : Product  Multiplication=Matrix(*)
  S-R Flip-Flop : simulink_extras/Flip Flops/S-R Flip-Flop  initial_condition=0
  Scope1 : Scope
  Scope2 : Scope
  Scope3 : Scope
  Stop Simulation : Stop
  To Workspace3 : ToWorkspace  VariableName=plaque_touche_butee  SampleTime=-1
      settings: MaxDataPoints=1
  Vector Concatenate : Concatenate  NumInputs=3  Mode=Multidimensional array
  wires:
  z/1 -> Vector Concatenate/3
  theta/1 -> Vector Concatenate/2
  phi/1 -> Vector Concatenate/1
  Constant/1 -> Product/1
  Vector Concatenate/1 -> Product/2
  Product/1 -> Demux/1
  Demux/1 -> Detection angle plus 5 degree/1(distance A), Scope1/1
  Demux/2 -> Detection angle plus 5 degree/2(distance B), Scope2/1
  Demux/3 -> Detection angle plus 5 degree/3(distance C), Scope3/1
  Detection angle plus 5 degree/1(detection butee) -> S-R Flip-Flop/1
  Constant1/1 -> S-R Flip-Flop/2
  S-R Flip-Flop/1 -> Stop Simulation/1, To Workspace3/1

== system SA_decouple_angles/ModeleNonLineaire/Subsystem/ToForce ==
  I : Inport
  Z : Inport  Port=2
  Add35 : Sum
  Divide2 : Product  Inputs=*/
  Subsystem : Subsystem
  Subsystem1 : Subsystem
  Force : Outport
  wires:
  Subsystem1/1(Out1) -> Divide2/1
  Z/1 -> Subsystem/1(In1)
  Subsystem/2(Out2) -> Divide2/2
  Divide2/1 -> Add35/1
  Add35/1 -> Force/1
  I/1 -> Subsystem1/1(In1)
  Subsystem/1(Out1) -> Add35/2

== system SA_decouple_angles/ModeleNonLineaire/Subsystem/ToForce1 ==
  I : Inport
  Z : Inport  Port=2
  Add35 : Sum
  Divide2 : Product  Inputs=*/
  Subsystem : Subsystem
  Subsystem1 : Subsystem
  Force : Outport
  wires:
  Subsystem1/1(Out1) -> Divide2/1
  Z/1 -> Subsystem/1(In1)
  Subsystem/2(Out2) -> Divide2/2
  Divide2/1 -> Add35/1
  Add35/1 -> Force/1
  I/1 -> Subsystem1/1(In1)
  Subsystem/1(Out1) -> Add35/2

== system SA_decouple_angles/ModeleNonLineaire/Subsystem/ToForce2 ==
  I : Inport
  Z : Inport  Port=2
  Add35 : Sum
  Divide2 : Product  Inputs=*/
  Subsystem : Subsystem
  Subsystem1 : Subsystem
  Force : Outport
  wires:
  Subsystem1/1(Out1) -> Divide2/1
  Z/1 -> Subsystem/1(In1)
  Subsystem/2(Out2) -> Divide2/2
  Divide2/1 -> Add35/1
  Add35/1 -> Force/1
  I/1 -> Subsystem1/1(In1)
  Subsystem/1(Out1) -> Add35/2

== system SA_decouple_angles/Asservissements/Subsystem/Comp phi/Double_AvPh ==
  signal_in : Inport
  AvPh : TransferFcn  Numerator=num_AvPh_SA8  Denominator=den_AvPh_SA8
  Ka : Gain  Gain=Ka_SA8
  signal_out : Outport
  wires:
  signal_in/1 -> Ka/1
  Ka/1 -> AvPh/1
  AvPh/1 -> signal_out/1

== system SA_decouple_angles/Asservissements/Subsystem/Comp theta/Double_AvPh ==
  signal_in : Inport
  AvPh : TransferFcn  Numerator=num_AvPh_SA8  Denominator=den_AvPh_SA8
  Ka : Gain  Gain=Ka_SA8
  signal_out : Outport
  wires:
  signal_in/1 -> Ka/1
  Ka/1 -> AvPh/1
  AvPh/1 -> signal_out/1

== system SA_decouple_angles/Asservissements/Subsystem/Comp z (methode 1)/Double AvPh ==
  in : Inport
  Comp simple AvPh : TransferFcn  Numerator=num_av_SA91  Denominator=den_av_SA91
  Comp simple AvPh1 : TransferFcn  Numerator=num_av_SA91  Denominator=den_av_SA91
  Gain : Gain  Gain=Ka_av_SA91
  out : Outport
  wires:
  Comp simple AvPh/1 -> Comp simple AvPh1/1
  Gain/1 -> Comp simple AvPh/1
  Comp simple AvPh1/1 -> out/1
  in/1 -> Gain/1

== system SA_decouple_angles/Asservissements/Subsystem/Comp z (methode 1)/Simple AvPh ==
  In1 : Inport
  Comp RePh : TransferFcn  Numerator=num_re_SA91  Denominator=den_re_SA91
  Gain : Gain  Gain=Kr_SA91
  Out1 : Outport
  wires:
  Gain/1 -> Comp RePh/1
  Comp RePh/1 -> Out1/1
  In1/1 -> Gain/1

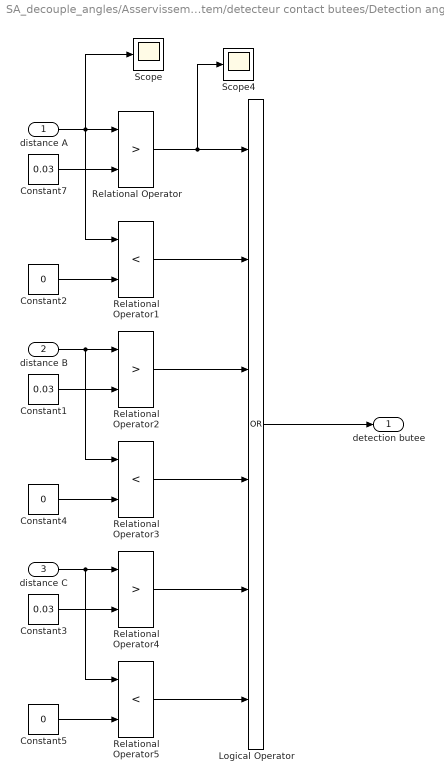
== system SA_decouple_angles/Asservissements/Subsystem/detecteur contact butees/Detection angle plus 5 degree ==
  distance A : Inport
  distance B : Inport  Port=2
  distance C : Inport  Port=3
  Constant1 : Constant  Value=0.03  OutDataTypeStr=double
  Constant2 : Constant  Value=0  OutDataTypeStr=double
  Constant3 : Constant  Value=0.03  OutDataTypeStr=double
  Constant4 : Constant  Value=0  OutDataTypeStr=double
  Constant5 : Constant  Value=0  OutDataTypeStr=double
  Constant7 : Constant  Value=0.03  OutDataTypeStr=double
  Logical Operator : Logic  Operator=OR  Inputs=6  AllPortsSameDT=off  OutDataTypeStr=boolean
  Relational Operator : RelationalOperator  Operator=>  OutDataTypeStr=boolean
  Relational Operator1 : RelationalOperator  Operator=<  OutDataTypeStr=boolean
  Relational Operator2 : RelationalOperator  Operator=>  OutDataTypeStr=boolean
  Relational Operator3 : RelationalOperator  Operator=<  OutDataTypeStr=boolean
  Relational Operator4 : RelationalOperator  Operator=>  OutDataTypeStr=boolean
  Relational Operator5 : RelationalOperator  Operator=<  OutDataTypeStr=boolean
  Scope : Scope
  Scope4 : Scope
  detection butee : Outport
  wires:
  distance A/1 -> Scope/1, Relational Operator1/1, Relational Operator/1
  Constant7/1 -> Relational Operator/2
  Constant2/1 -> Relational Operator1/2
  Relational Operator/1 -> Scope4/1, Logical Operator/1
  Relational Operator1/1 -> Logical Operator/2
  distance B/1 -> Relational Operator3/1, Relational Operator2/1
  Constant1/1 -> Relational Operator2/2
  Constant4/1 -> Relational Operator3/2
  Relational Operator2/1 -> Logical Operator/3
  Relational Operator3/1 -> Logical Operator/4
  distance C/1 -> Relational Operator5/1, Relational Operator4/1
  Constant3/1 -> Relational Operator4/2
  Constant5/1 -> Relational Operator5/2
  Relational Operator4/1 -> Logical Operator/5
  Relational Operator5/1 -> Logical Operator/6
  Logical Operator/1 -> detection butee/1

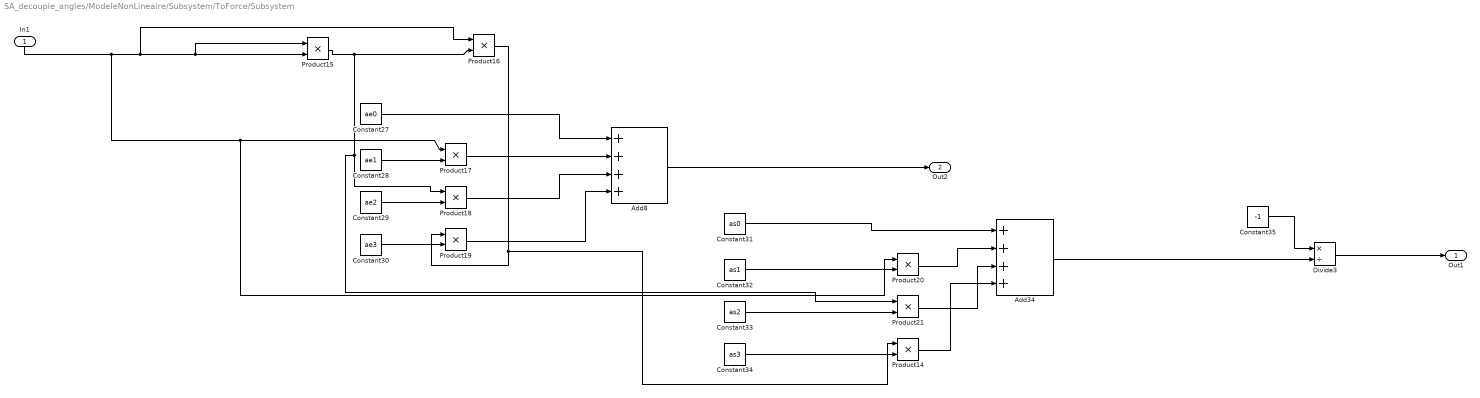
== system SA_decouple_angles/ModeleNonLineaire/Subsystem/ToForce/Subsystem ==
  In1 : Inport
  Add34 : Sum  Inputs=++++
  Add8 : Sum  Inputs=++++
  Constant27 : Constant  Value=ae0
  Constant28 : Constant  Value=ae1
  Constant29 : Constant  Value=ae2
  Constant30 : Constant  Value=ae3
  Constant31 : Constant  Value=as0
  Constant32 : Constant  Value=as1
  Constant33 : Constant  Value=as2
  Constant34 : Constant  Value=as3
  Constant35 : Constant  Value=-1
  Divide3 : Product  Inputs=*/
  Product{14..21} (8 alike) : Product
  Out1 : Outport
  Out2 : Outport  Port=2
  wires:
  In1/1 -> Product20/1, Product17/1, Product16/1, Product15/1, Product15/2
  Constant28/1 -> Product17/2
  Constant30/1 -> Product19/2
  Constant29/1 -> Product18/2
  Product15/1 -> Product21/1, Product18/1, Product16/2
  Product16/1 -> Product19/1, Product14/1
  Constant27/1 -> Add8/1
  Product17/1 -> Add8/2
  Product18/1 -> Add8/3
  Product19/1 -> Add8/4
  Add8/1 -> Out2/1
  Constant34/1 -> Product14/2
  Constant32/1 -> Product20/2
  Constant33/1 -> Product21/2
  Product20/1 -> Add34/2
  Product21/1 -> Add34/3
  Product14/1 -> Add34/4
  Constant31/1 -> Add34/1
  Add34/1 -> Divide3/2
  Constant35/1 -> Divide3/1
  Divide3/1 -> Out1/1

== system SA_decouple_angles/ModeleNonLineaire/Subsystem/ToForce/Subsystem1 ==
  In1 : Inport
  Abs1 : Abs
  Add7 : Sum
  Constant26 : Constant  Value=be1
  Product11 : Product
  Product12 : Product
  Product13 : Product
  Sign1 : Signum
  Out1 : Outport
  wires:
  In1/1 -> Abs1/1, Sign1/1, Product11/2, Product11/1
  Constant26/1 -> Product12/1
  Abs1/1 -> Product12/2
  Product12/1 -> Add7/1
  Product11/1 -> Add7/2
  Add7/1 -> Product13/2
  Product13/1 -> Out1/1
  Sign1/1 -> Product13/1

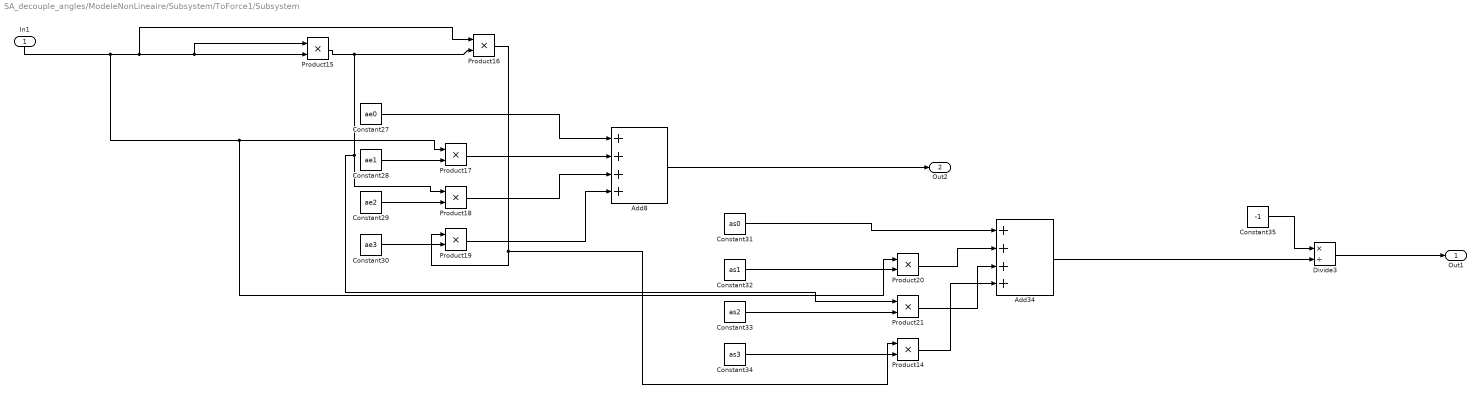
== system SA_decouple_angles/ModeleNonLineaire/Subsystem/ToForce1/Subsystem ==
  In1 : Inport
  Add34 : Sum  Inputs=++++
  Add8 : Sum  Inputs=++++
  Constant27 : Constant  Value=ae0
  Constant28 : Constant  Value=ae1
  Constant29 : Constant  Value=ae2
  Constant30 : Constant  Value=ae3
  Constant31 : Constant  Value=as0
  Constant32 : Constant  Value=as1
  Constant33 : Constant  Value=as2
  Constant34 : Constant  Value=as3
  Constant35 : Constant  Value=-1
  Divide3 : Product  Inputs=*/
  Product{14..21} (8 alike) : Product
  Out1 : Outport
  Out2 : Outport  Port=2
  wires:
  In1/1 -> Product20/1, Product17/1, Product16/1, Product15/1, Product15/2
  Constant28/1 -> Product17/2
  Constant30/1 -> Product19/2
  Constant29/1 -> Product18/2
  Product15/1 -> Product21/1, Product18/1, Product16/2
  Product16/1 -> Product19/1, Product14/1
  Constant27/1 -> Add8/1
  Product17/1 -> Add8/2
  Product18/1 -> Add8/3
  Product19/1 -> Add8/4
  Add8/1 -> Out2/1
  Constant34/1 -> Product14/2
  Constant32/1 -> Product20/2
  Constant33/1 -> Product21/2
  Product20/1 -> Add34/2
  Product21/1 -> Add34/3
  Product14/1 -> Add34/4
  Constant31/1 -> Add34/1
  Add34/1 -> Divide3/2
  Constant35/1 -> Divide3/1
  Divide3/1 -> Out1/1

== system SA_decouple_angles/ModeleNonLineaire/Subsystem/ToForce1/Subsystem1 ==
  In1 : Inport
  Abs1 : Abs
  Add7 : Sum
  Constant26 : Constant  Value=be1
  Product11 : Product
  Product12 : Product
  Product13 : Product
  Sign1 : Signum
  Out1 : Outport
  wires:
  In1/1 -> Abs1/1, Sign1/1, Product11/2, Product11/1
  Constant26/1 -> Product12/1
  Abs1/1 -> Product12/2
  Product12/1 -> Add7/1
  Product11/1 -> Add7/2
  Add7/1 -> Product13/2
  Product13/1 -> Out1/1
  Sign1/1 -> Product13/1

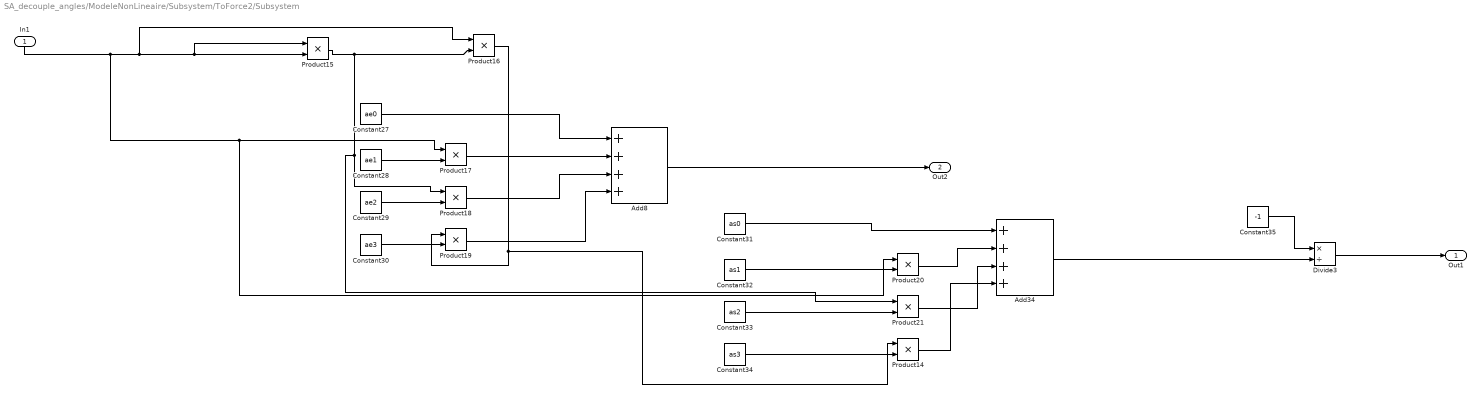
== system SA_decouple_angles/ModeleNonLineaire/Subsystem/ToForce2/Subsystem ==
  In1 : Inport
  Add34 : Sum  Inputs=++++
  Add8 : Sum  Inputs=++++
  Constant27 : Constant  Value=ae0
  Constant28 : Constant  Value=ae1
  Constant29 : Constant  Value=ae2
  Constant30 : Constant  Value=ae3
  Constant31 : Constant  Value=as0
  Constant32 : Constant  Value=as1
  Constant33 : Constant  Value=as2
  Constant34 : Constant  Value=as3
  Constant35 : Constant  Value=-1
  Divide3 : Product  Inputs=*/
  Product{14..21} (8 alike) : Product
  Out1 : Outport
  Out2 : Outport  Port=2
  wires:
  In1/1 -> Product20/1, Product17/1, Product16/1, Product15/1, Product15/2
  Constant28/1 -> Product17/2
  Constant30/1 -> Product19/2
  Constant29/1 -> Product18/2
  Product15/1 -> Product21/1, Product18/1, Product16/2
  Product16/1 -> Product19/1, Product14/1
  Constant27/1 -> Add8/1
  Product17/1 -> Add8/2
  Product18/1 -> Add8/3
  Product19/1 -> Add8/4
  Add8/1 -> Out2/1
  Constant34/1 -> Product14/2
  Constant32/1 -> Product20/2
  Constant33/1 -> Product21/2
  Product20/1 -> Add34/2
  Product21/1 -> Add34/3
  Product14/1 -> Add34/4
  Constant31/1 -> Add34/1
  Add34/1 -> Divide3/2
  Constant35/1 -> Divide3/1
  Divide3/1 -> Out1/1

== system SA_decouple_angles/ModeleNonLineaire/Subsystem/ToForce2/Subsystem1 ==
  In1 : Inport
  Abs1 : Abs
  Add7 : Sum
  Constant26 : Constant  Value=be1
  Product11 : Product
  Product12 : Product
  Product13 : Product
  Sign1 : Signum
  Out1 : Outport
  wires:
  In1/1 -> Abs1/1, Sign1/1, Product11/2, Product11/1
  Constant26/1 -> Product12/1
  Abs1/1 -> Product12/2
  Product12/1 -> Add7/1
  Product11/1 -> Add7/2
  Add7/1 -> Product13/2
  Product13/1 -> Out1/1
  Sign1/1 -> Product13/1
